simulink model "E"  (R2020a)
settings: Solver=VariableStepAuto  StartTime=0.0  StopTime=10.0  RelTol=1e-3
settings Model: Creator=Admin  LastModifiedBy=Admin

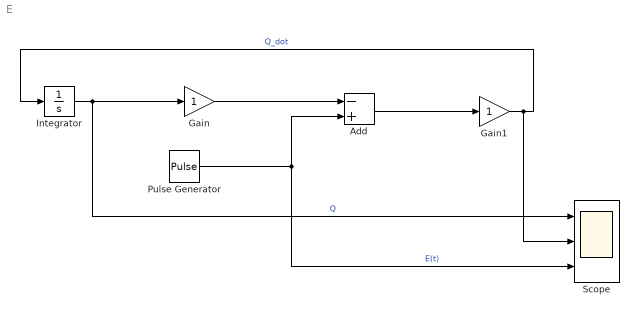
== system E ==
  Add : Sum  Inputs=-+
  Gain : Gain
  Gain1 : Gain
  Integrator : Integrator
  Pulse Generator : DiscretePulseGenerator  PulseType=Time based  Period=10  PulseWidth=5
  Scope : Scope  NumInputPorts=3
  wires:
  Integrator/1 -> Scope/1, Gain/1  "Q"
  Gain/1 -> Add/1
  Add/1 -> Gain1/1
  Gain1/1 -> Scope/2, Integrator/1  "Q_dot"
  Pulse Generator/1 -> Add/2, Scope/3  "E(t)"
